simulink model "SAC_RL_env (no DEEN, orig)"  (R2025b)
settings: Solver=ode4  StartTime=0.0  StopTime=400  FixedStep=0.005  RelTol=1e-3  EnableMultiTasking=on
values from neighbouring files (symbols this model uses):
  dyn_obs = struct('p0', cell(1, num_dyn_obs), 'v', cell(1, num_dyn_obs), 'radius', cell(1, num_dyn_obs))    [genera_ostacoli_dinamici.m]    (also in visualizza_raggi_completo.m = scenario.dynamic_obstacles)
  initialGainsMultiplier = 15    [init_rl.m]    (also in report_agent.m; test.m; test_agent.m; train.m)
  is_validation = env.isValidation    [CustomSimulinkEnv.m]    (also in get_RL_env.m = evalin('base', 'is_validation'))
  logging = true    [train.m]    (also in train_agent.m; train_agent_precedente.m)
  max_angular_vel = double(pi)    [get_RL_env.m]
  max_deviazione_pos = 100    [get_RL_env.m]
  max_deviazione_vel = 20    [get_RL_env.m]
  max_distanza_goal = double(norm(initial_pos - scenario.map.q_goal))    [get_RL_env.m]
  max_vel = 30    [get_RL_env.m]
  num_rays = size(lidar_scan, 2)    [visualizza_raggi.m]
  tolleranza_goal = 2    [get_RL_env.m]
  Ts = 0.1    [init_rl.m]    (also in report_agent.m; test.m; test_agent.m; train.m)
undefined symbols (not defined in the file or in its folder): angControlTuning, angRateControlTuning, bounds, Controller, decyear, DiscIntNeverNeededParam, DroneMass, Dz, Gravity, initialConditions, Iz, leapyear, logPath_num, logPathValid_num, Nz, pos_goal, posControlTuning, Pz, startFlightTime, tunePositionController, UAVSampleTime, Vehicle, velControlTuning
libraries: slpidlib x14, slctrl_autotuning x8, sharedutil x4, matrix_library x4, aerolibconvert2 x3, aerolibatmos2 x2, aerolibgravity2 x2, shared6dof x2, aerolibasang x2, sensorinslib x2, deeplib x1, rllib x1
(part 5 of 5)

== matlab function SAC_RL_env (no DEEN, orig)/Inner Loop and Plant Model/High-FidelityModel/MATLAB Function2 ==
  data: distanza_goal input; isdone input; flags input; logging parameter; logPath_num parameter size=[1 250]; t input; reward_curr input; rewards input; is_validation parameter; logPathValid_num parameter
function logging_function(distanza_goal, isdone, flags, logging, logPath_num, t, reward_curr, rewards, is_validation, logPathValid_num)
    coder.extrinsic('fopen', 'fprintf', 'fclose', 'disp');
    persistent total_steps
    persistent total_reward
    persistent total_rewards
    
    if isempty(total_steps)
        total_steps = 0;
        total_reward = 0;
        total_rewards = [0 0 0 0 0];
    end
    
    if t == 0
        total_steps = 0;
        total_reward = 0;
        total_rewards = [0 0 0 0 0];
        return
    end
    
    total_steps = total_steps + 1;
    total_reward = total_reward + reward_curr;

    for i=1:length(rewards)
        total_rewards(i) = total_rewards(i) + rewards(i);
    end
    
    if logging
        if isdone
            distanza_goal = double(distanza_goal);
            
            fuori_traiettoria = flags(1);
            schianto_terra    = flags(2);
            collisione        = flags(3);
            traguardo_raggiunto = flags(4);
            
            % Estrazione percorso
            logPath = strtrim(char(logPath_num));

            if is_validation
                logPath = strtrim(char(logPathValid_num));
            end
            
            % PRE-ALLOCAZIONE FONDAMENTALE PER SIMULINK CODER
            fileID = -1; 
            fileID = fopen(logPath, 'a');
            
            if fileID ~= -1
                if schianto_terra
                    fprintf(fileID, 'Step: %d | Rwd: %.2f | Distanza goal: %.2f | Motivo: Schianto a terra\n', int32(total_steps), double(total_reward), distanza_goal);
                elseif collisione
                    fprintf(fileID, 'Step: %d | Rwd: %.2f | Distanza goal: %.2f | Motivo: Collisione ostacolo\n', int32(total_steps), double(total_reward), distanza_goal);
                elseif fuori_traiettoria
                    fprintf(fileID, 'Step: %d | Rwd: %.2f | Distanza goal: %.2f | Motivo: Deviazione eccessiva\n', int32(total_steps), double(total_reward), distanza_goal);
                elseif traguardo_raggiunto
                    fprintf(fileID, 'Step: %d | Rwd: %.2f | Distanza goal: %.2f | Motivo: TRAGUARDO RAGGIUNTO!\n', int32(total_steps), double(total_reward), distanza_goal);
                end
                fprintf(fileID, 'azioni: %f | ostacoli: %f | posizione: %f | velocita: %f | progresso: %f\n\n', total_rewards(1), total_rewards(2), total_rewards(3), total_rewards(4), total_rewards(5));
                fclose(fileID);
            else

                disp(' ');
                disp('!!! ERRORE SIMULINK !!! Impossibile creare/aprire il file!');
                disp(['Percorso tentato: ', logPath]);
                disp('Controlla se il percorso è corretto o se OneDrive sta bloccando il file.');
                disp(' ');
            end
        end
    end
end

== matlab function SAC_RL_env (no DEEN, orig)/Inner Loop and Plant Model/High-FidelityModel/Errors extractor/Errors normalization ==
  data: errors input; errors_normalized output; max_deviazione_pos parameter; max_deviazione_vel parameter
function errors_normalized = errors_normalization(errors, max_deviazione_pos, max_deviazione_vel)
    e_pos = errors(1:3);
    e_vel = errors(4:6);

    errors_normalized = errors;

    % % Normalizzazione degli errori nel range [0, 1]
    e_pos_norm = e_pos / max_deviazione_pos;
    e_vel_norm = e_vel / max_deviazione_vel;

    e_pos_norm = max(min(e_pos_norm, 1.0), -1.0);
    e_vel_norm = max(min(e_vel_norm, 1.0), -1.0);

    errors_normalized(1:3) = e_pos_norm;
    errors_normalized(4:6) = e_vel_norm;
end

== matlab function SAC_RL_env (no DEEN, orig)/Inner Loop and Plant Model/High-FidelityModel/State normalization ==
  data: distanza_goal_norm output; distanza_goal input; state input; state_norm output; max_angular_vel parameter; max_vel parameter; max_distanza_goal parameter
function [distanza_goal_norm, state_norm] = state_normalization(distanza_goal, state, max_angular_vel, max_vel, max_distanza_goal)
    vel = state(1:3);
    angular_vel = state(4:6);

    state_norm = state;

    vel_norm = vel / max_vel;
    angular_vel = angular_vel / max_angular_vel;

    vel_norm = max(min(vel_norm, 1.0), -1.0);
    angular_vel = max(min(angular_vel, 1.0), -1.0);

    state_norm(1:3) = vel_norm;
    state_norm(4:6) = angular_vel;

    distanza_goal_norm = distanza_goal / max_distanza_goal;
end

== matlab function SAC_RL_env (no DEEN, orig)/Inner Loop and Plant Model/High-FidelityModel/Input_Normalization ==
  data: raggi_lidar_t input; stato_t input; Input_Normalization output; motori input; raggi_lidar_t_succ input; stato_t_succ input
function Input_Normalization = prepara_input_deen(raggi_lidar_t, stato_t, motori, raggi_lidar_t_succ, stato_t_succ)
    %#codegen
    % Direttiva per la generazione di codice C ultra-rapido in Simulink
    
    % Inizializzazione delle variabili in memoria statica (RAM)
    persistent media_deen std_deen
    
    if isempty(media_deen)
        % coder.load "cuoce" i dati nel blocco C al momento della compilazione
        % Zero latenza di lettura dal disco durante la simulazione
        dati = coder.load('statistiche_deen.mat');
        
        % Pre-formattazione rigorosa in vettori riga (1x536)
        media_deen = dati.mean_train(:)';
        std_deen = dati.std_train(:)';
    end
    
    % --- OPZIONALE: GESTIONE ASSE Z (NED -> Standard) ---
    % Se la componente Vz (il 3° elemento dello stato) arriva grezza da Simulink (NED), 
    % decommenta queste due righe per invertirla al volo senza creare nuove variabili.
    % stato_t(3) = -stato_t(3);
    % stato_t_succ(3) = -stato_t_succ(3);
    % ----------------------------------------------------
    
    % 1. Concatenazione ad altissime prestazioni. 
    % L'operatore (:) seguito da ' forza istantaneamente qualsiasi input a vettore riga,
    % proteggendoti da errori di dimensione ("dimension mismatch") senza usare cicli o if.
    stato_grezzo = [raggi_lidar_t(:)', stato_t(:)', motori(:)', raggi_lidar_t_succ(:)', stato_t_succ(:)'];
    
    % 2. Normalizzazione Vettoriale Z-Score
    % Questa singola riga esegue 536 sottrazioni e 536 divisioni in parallelo,
    % sfruttando al massimo il processore tramite l'operatore ./ (element-wise)
    Input_Normalization = (stato_grezzo - media_deen) ./ std_deen;
    
end

== matlab function SAC_RL_env (no DEEN, orig)/Inner Loop and Plant Model/High-FidelityModel/Control System/Controller/Position Controller/Position error transformation (Earth to Body frame) ==
  data: yaw input; xy_err_earth input; xy_err_body output
function xy_err_body = LTP2B2D(yaw,xy_err_earth)

transformation = [cos(yaw), sin(yaw); -sin(yaw),  cos(yaw)];
xy_err_body = transformation * xy_err_earth;


end

== matlab function SAC_RL_env (no DEEN, orig)/Inner Loop and Plant Model/High-FidelityModel/Control System/Controller/Position Controller/Velocity error transformation (Earth to Body frame) ==
  data: yaw input; xy_err_earth input; xy_err_body output
function xy_err_body = LTP2B2D(yaw,xy_err_earth)

transformation = [cos(yaw), sin(yaw); -sin(yaw),  cos(yaw)];
xy_err_body = transformation * xy_err_earth;


end

== matlab function SAC_RL_env (no DEEN, orig)/Inner Loop and Plant Model/High-FidelityModel/Control System/Controller/Yaw Controller/MATLAB Function ==
  data: u input; y output single
function y = wrapYaw(u)
%u error in rad in -2pi to 2pi

if (u>pi)
    y = single(u-2*pi);
elseif(u<-pi)
    y = single(u +2*pi);
else
    y=single(u);
end

== matlab function SAC_RL_env (no DEEN, orig)/Inner Loop and Plant Model/High-FidelityModel/Control System/Controller/Yaw Controller/MATLAB Function1 ==
  data: u input; y output
function y = wrapYaw(u)
%u error in rad in -2pi to 2pi

if (u>pi)
    y = u-2*pi;
elseif(u<-pi)
    y = u +2*pi;
else
    y=u;
end

== matlab function SAC_RL_env (no DEEN, orig)/Inner Loop and Plant Model/High-FidelityModel/Control System/Controller/Position Controller/Velocity error transformation (Earth to Body frame)1 ==
  data: yaw input; xy_err_earth input; xy_err_body output
function xy_err_body = LTP2B2D(yaw,xy_err_earth)

transformation = [cos(yaw), sin(yaw); -sin(yaw),  cos(yaw)];
xy_err_body = transformation * xy_err_earth;


end

== matlab function SAC_RL_env (no DEEN, orig)/Inner Loop and Plant Model/High-FidelityModel/State and Rays extractor/MATLAB Function ==
  data: pos_drone input; lidar_scan output double; bounds parameter; dyn_obs parameter; t input; num_rays parameter
function lidar_scan = estrai_lidar_scan(pos_drone, bounds, dyn_obs, t, num_rays)
    % Parametri del sensore
    max_range = 20.0; % Raggio massimo in metri
    % Aumentiamo i raggi: 256 o 512 sono buoni compromessi per RL in 3D
    
    % === 1. GENERAZIONE DIREZIONI RAGGI (SFERA DI FIBONACCI) ===
    % Genera vettori direzione unitari uniformemente distribuiti in 3D.
    indices = 0:(num_rays - 1);
    phi = pi * (3 - sqrt(5)); % Angolo aureo in radianti
    
    % La Z varia uniformemente da 1 (Polo Nord) a -1 (Polo Sud)
    z = 1 - (indices ./ (num_rays - 1)) .* 2; 
    
    % Raggio sul piano XY per l'altezza Z corrente
    raggio_xy = sqrt(1 - z.^2); 
    
    % Angolo di rotazione attorno all'asse Z
    theta = phi .* indices;      
    
    % Calcolo componenti X e Y
    x = cos(theta) .* raggio_xy;
    y = sin(theta) .* raggio_xy;
    
    % Matrice 3 x num_rays di vettori direzione unitari
    dirs = double([x; y; z]); 
    
    % Inizializza l'array delle misurazioni alla distanza massima
    lidar_scan = max_range * ones(1, num_rays, 'double');

    pos_drone = double(pos_drone);

    % === 1.5 ADATTAMENTO FORMATO BOUNDS (STRUCT o MATRICE) ===
    % Questo blocco rende la funzione universale per qualsiasi tipo di mappa
    if isstruct(bounds)
        b_xmin = bounds.x_min; b_xmax = bounds.x_max;
        b_ymin = bounds.y_min; b_ymax = bounds.y_max;
        b_zmin = bounds.z_min; b_zmax = bounds.z_max;
    else
        % Se bounds è una matrice Nx6 (es. map.v)
        if size(bounds, 2) >= 6
            % Controlla se il formato è [xmin, xmax, ymin, ymax, ...] o [xmin, ymin, zmin, xmax, ...]
            if bounds(1,2) > bounds(1,1) && bounds(1,4) > bounds(1,3)
                b_xmin = bounds(:,1); b_xmax = bounds(:,2);
                b_ymin = bounds(:,3); b_ymax = bounds(:,4);
                b_zmin = bounds(:,5); b_zmax = bounds(:,6);
            else
                b_xmin = bounds(:,1); b_xmax = bounds(:,4);
                b_ymin = bounds(:,2); b_ymax = bounds(:,5);
                b_zmin = bounds(:,3); b_zmax = bounds(:,6);
            end
        else
            b_xmin = []; b_xmax = []; b_ymin = []; b_ymax = []; b_zmin = []; b_zmax = [];
        end
    end

    % === 2. INTERSEZIONE CON OSTACOLI STATICI (PALAZZI - SLAB METHOD) ===
    if ~isempty(b_xmin)
        % Uso i vettori estratti al passo 1.5
        vicini_idx = find(~(b_xmax < pos_drone(1)-max_range | b_xmin > pos_drone(1)+max_range | ...
                            b_ymax < pos_drone(2)-max_range | b_ymin > pos_drone(2)+max_range | ...
                            b_zmax < pos_drone(3)-max_range | b_zmin > pos_drone(3)+max_range));

    % === 2. INTERSEZIONE CON OSTACOLI STATICI (PALAZZI - SLAB METHOD) ===
    vicini_idx = find(~(bounds.x_max < pos_drone(1)-max_range | bounds.x_min > pos_drone(1)+max_range | ...
                        bounds.y_max < pos_drone(2)-max_range | bounds.y_min > pos_drone(2)+max_range | ...
                        bounds.z_max < pos_drone(3)-max_range | bounds.z_min > pos_drone(3)+max_range));
                        
    if ~isempty(vicini_idx)
        % Precalcola i reciproci delle direzioni per lo Slab Method.
        % L'aggiunta di 1e-8 previene divisioni per zero quando un raggio 
        % è perfettamente parallelo a un asse.
        inv_dirs = 1 ./ (dirs + 1e-8); 
        
        for i = 1:length(vicini_idx)
            idx = vicini_idx(i);
            
            % Limiti del bounding box corrente
            b_min = [bounds.x_min(idx); bounds.y_min(idx); bounds.z_min(idx)];
            b_max = [bounds.x_max(idx); bounds.y_max(idx); bounds.z_max(idx)];
            
            % Calcola i tempi di intersezione con i piani min e max per gli assi XYZ
            % (Operazione matriciale 3 x num_rays)
            t0 = (b_min - pos_drone(:)) .* inv_dirs; 
            t1 = (b_max - pos_drone(:)) .* inv_dirs; 
            
            % tmin è il tempo di ingresso nel piano, tmax l'uscita per ogni asse
            tmin = min(t0, t1); 
            tmax = max(t0, t1); 
            
            % Il raggio entra nel box quando ha superato TUTTI E TRE i piani min
            t_enter = max(tmin, [], 1); % Estrae il max lungo le colonne (1 x num_rays)
            
            % Il raggio esce dal box appena supera UNO DEI TRE piani max
            t_exit = min(tmax, [], 1);  % Estrae il min lungo le colonne (1 x num_rays)
            
            % Condizione di intersezione Ray-AABB:
            % 1. Entra prima di uscire (t_enter <= t_exit)
            % 2. L'uscita è davanti al drone (t_exit > 0)
            hit_mask = (t_enter <= t_exit) & (t_exit > 0);
            
            if any(hit_mask)
                hitting_rays = find(hit_mask);
                for j = 1:length(hitting_rays)
                    r_idx = hitting_rays(j);
                    
                    % Se il drone è all'interno del palazzo, t_enter è negativo.
                    % In tal caso, la distanza di impatto è 0 (schianto istantaneo).
                    if t_enter(r_idx) > 0
                        d_imp = t_enter(r_idx);
                    else
                        d_imp = 0; 
                    end
                    
                    % Sovrascrivi se questo palazzo è più vicino di altri ostacoli già visti
                    if d_imp < lidar_scan(r_idx)
                        lidar_scan(r_idx) = d_imp;
                    end
                end
            end
        end
    end

    % === 3. INTERSEZIONE CON OSTACOLI DINAMICI (SFERE) ===
    if ~isempty(dyn_obs)
        for k = 1:length(dyn_obs)

            %Calcola la posizione attuale dell'ostacolo: P(t) = P0 + V*t
            centro_sfera = dyn_obs(k).p0 + dyn_obs(k).v * t;
            raggio_sfera = dyn_obs(k).radius;
            
            % Vettore dal drone al centro della sfera (3x1)
            v = centro_sfera(:) - pos_drone(:);
            
            % Proiezione vettorializzata: dot product tra 'v' e tutti i raggi 'dirs'
            proj = v' * dirs; 
            
            % Consideriamo solo i raggi per cui la sfera è "in avanti"
            valid_idx = proj > 0;
            
            if any(valid_idx)
                % Calcolo distanza ortogonale per i raggi validi
                distanza_ortogonale_sq = dot(v, v) - proj(valid_idx).^2;
                
                % Trova quali raggi hanno colpito la sfera
                hit_idx = distanza_ortogonale_sq <= raggio_sfera^2;
                
                if any(hit_idx)
                    actual_rays = find(valid_idx);
                    hitting_rays = actual_rays(hit_idx);
                    
                    proj_hits = proj(hitting_rays);
                    dist_ort_sq_hits = distanza_ortogonale_sq(hit_idx);
                    distanza_impatto = proj_hits - sqrt(raggio_sfera^2 - dist_ort_sq_hits);
                    
                    for i = 1:length(hitting_rays)
                        r_idx = hitting_rays(i);
                        d_imp = distanza_impatto(i);
                        if d_imp > 0 && d_imp < lidar_scan(r_idx)
                            lidar_scan(r_idx) = d_imp;
                        end
                    end
                end
            end
        end
    end

    % === 4. INTERSEZIONE CON IL TERRENO (PIANO Z = -1) ===
    % Consideriamo solo i raggi che puntano verso il basso (z < 0)
    downward_rays = dirs(3,:) < 0;

    if any(downward_rays)
        % Calcoliamo l'intersezione con il piano z=-0.5
        % L'equazione del piano è z = -0.5
        % Per un raggio con direzione (dx, dy, dz) e origine (x0, y0, z0):
        % z0 + t*dz = -0.5 => t = (-0.5 - z0)/dz
        t_ground = (-0.5 - pos_drone(3)) ./ dirs(3, downward_rays);

        % Filtriamo solo le intersezioni valide (t > 0)
        valid_ground = t_ground > 0;

        if any(valid_ground)
            ground_rays = find(downward_rays);
            valid_ground_rays = ground_rays(valid_ground);

            % Calcoliamo le distanze di impatto
            d_imp = t_ground(valid_ground);

            % Aggiorniamo le misurazioni lidar
            for i = 1:length(valid_ground_rays)
                r_idx = valid_ground_rays(i);
                if d_imp(i) < lidar_scan(r_idx)
                    lidar_scan(r_idx) = d_imp(i);
                end
            end
        end
    end
    
    % Normalizzazione
    % L'output è un array flat [1 x num_rays] con valori nel range [0, 1]
    lidar_scan = double(lidar_scan) / max_range;
end

== matlab function SAC_RL_env (no DEEN, orig)/Inner Loop and Plant Model/High-FidelityModel/Plant Model/Bus setup/Generate GPS Data/Scale and Assemble GPS Data /Embedded MATLAB Function1 ==
  data: cog output; Vn input; Ve input
function cog = getCOG(Vn, Ve)
% This block supports an embeddable subset of the MATLAB language.
% See the help menu for details. 

cog = atan2(Ve,Vn);
if cog < 0;
    cog = cog + 2*pi;
end

== matlab function SAC_RL_env (no DEEN, orig)/Inner Loop and Plant Model/High-FidelityModel with Autotuning/Control System/Controller/Position Controller/Position error transformation (Earth to Body frame) ==
  data: yaw input; xy_err_earth input; xy_err_body output
function xy_err_body = LTP2B2D(yaw,xy_err_earth)

transformation = [cos(yaw), sin(yaw); -sin(yaw),  cos(yaw)];
xy_err_body = transformation * xy_err_earth;


end

== matlab function SAC_RL_env (no DEEN, orig)/Inner Loop and Plant Model/High-FidelityModel/MATLAB Function ==
  data: tracking_error output; distanza_goal output; pos_curr input; isdone output; pos_des input; rays input; pos_goal parameter size=[1 3]; flags output; t input; max_deviazione_pos parameter; tolleranza_goal parameter
function [tracking_error, distanza_goal, isdone, flags] = check_terminal_state(pos_curr, pos_des, rays, pos_goal, t, max_deviazione_pos, tolleranza_goal)

    persistent raggio_drone
    persistent soglia_impatto
    persistent max_range_raggi

    if isempty(raggio_drone)
   
        raggio_drone = 0.5; % Ingombro fisico del drone in metri (30 cm)
        max_range_raggi = 20; % Lo stesso usato nel raycasting
        soglia_impatto = raggio_drone / max_range_raggi;
    end

    pos_goal = pos_goal';


    % Ignora forzatamente il primo loop (t = 0)
    if t == 0
        isdone = false;
        flags = [false, false, false, false];
        distanza_goal = double(norm(pos_curr - pos_goal));
        tracking_error = 0;
        return; % Esce immediatamente dalla funzione
    end
    
    % 1. Controllo Divergenza (Tracking Error)
    % Calcola la distanza euclidea tra la posizione attuale e quella desiderata
    tracking_error = double(norm(pos_curr - pos_des));
    fuori_traiettoria =  tracking_error > max_deviazione_pos;
    
    % 2. Controllo Altitudine (Schianto a terra)
    % Presumendo che pos_curr(3) sia l'altitudine (asse Z positivo verso l'alto)
    quota_minima = 0;
    schianto_terra = pos_curr(3) < quota_minima;
    
    % 3. Controllo Collisione tramite raggi LiDAR
    % Si valuta se l'ostacolo più vicino penetra il raggio fisico del drone
    collisione = false;
    if min(rays) <= soglia_impatto
        collisione = true;
    end

    % Controllo Traguardo Raggiunto
    distanza_goal = double(norm(pos_curr - pos_goal));
    traguardo_raggiunto = distanza_goal < tolleranza_goal;

    flags = [fuori_traiettoria, schianto_terra, collisione, traguardo_raggiunto];
    
    % L'episodio termina se si verifica ALMENO UNA di queste condizioni
    isdone = fuori_traiettoria | schianto_terra | collisione | traguardo_raggiunto;
    
end
